simulink model "controller"  (R2019b)
settings: Solver=FixedStepAuto  StartTime=0.0  StopTime=10.0  RelTol=1e-3
undefined symbols (not defined in the file or in its folder): DiscIntNeverNeededParam, k_simulazione_discreta, phi_p_setpoint, Ts
settings Model: Creator=AndreaCalegari  LastModifiedBy=AndreaCalegari

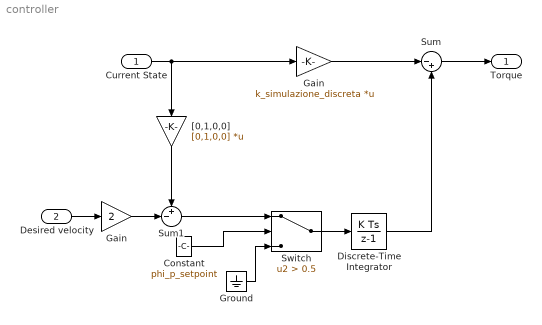
== system controller ==
  Current State : Inport  PortDimensions=4  SampleTime=Ts
  "Desired velocity " : Inport  Port=2  SampleTime=Ts
  Constant : Constant  Value=phi_p_setpoint
  Discrete-Time Integrator : DiscreteIntegrator  gainval=0.00227178510009537  SampleTime=Ts  ICPrevOutput=DiscIntNeverNeededParam  ICPrevScaledInput=DiscIntNeverNeededParam
  Gain : Gain  Gain=2
  "Gain " : Gain  Gain=k_simulazione_discreta  Multiplication=Matrix(K*u)
  Ground : Ground
  Sum : Sum  Inputs=|-+
  Sum1 : Sum  Inputs=+-|
  Switch : Switch  Criteria=u2 > Threshold  Threshold=0.5
  "[0,1,0,0]" : Gain  Gain=[0,1,0,0]  Multiplication=Matrix(K*u)
  Torque : Outport  SampleTime=Ts
  wires:
  Sum/1 -> Torque/1
  "[0,1,0,0]"/1 -> Sum1/1
  Sum1/1 -> Switch/1
  "Gain "/1 -> Sum/1
  Discrete-Time Integrator/1 -> Sum/2
  Current State/1 -> "Gain "/1, "[0,1,0,0]"/1
  Switch/1 -> Discrete-Time Integrator/1
  "Desired velocity "/1 -> Gain/1
  Constant/1 -> Switch/2
  Ground/1 -> Switch/3
  Gain/1 -> Sum1/2
